simulink model "MBD_Week2_Prob4"  (R2020a)
settings: Solver=ode15s  StartTime=0.0  StopTime=0.2  RelTol=1e-3
undefined symbols (not defined in the file or in its folder): Kd, Ki, Kp
settings Model: DataDictionary=Motor_Pos_DD.sldd  Creator=Noel Varghese  LastModifiedBy=Noel Varghese

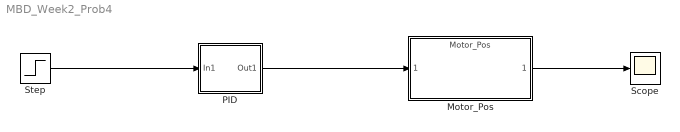
== system MBD_Week2_Prob4 ==
  Motor_Pos : ModelReference  ModelNameDialog=Motor_Pos  ModelReferenceVersion=1.4
  PID : Subsystem
  Scope : Scope
  Step : Step  Time=0  SampleTime=0
  wires:
  Motor_Pos/1 -> Scope/1
  Step/1 -> PID/1(In1)
  PID/1(Out1) -> Motor_Pos/1

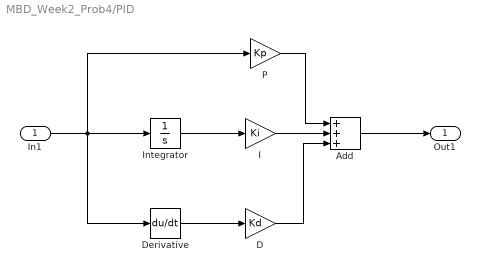
== system MBD_Week2_Prob4/PID ==
  In1 : Inport
  Add : Sum  Inputs=+++
  D : Gain  Gain=Kd
  Derivative : Derivative
  I : Gain  Gain=Ki
  Integrator : Integrator
  P : Gain  Gain=Kp
  Out1 : Outport
  wires:
  In1/1 -> Derivative/1, P/1, Integrator/1
  D/1 -> Add/3
  Add/1 -> Out1/1
  P/1 -> Add/1
  Derivative/1 -> D/1
  Integrator/1 -> I/1
  I/1 -> Add/2
